simulink library "AD_Snowman_Library"  (R2023b)
settings: Solver=VariableStepAuto  StartTime=0.0  StopTime=10.0  RelTol=1e-3
libraries: simulink x1, $bdroot x1
settings Model: LastModifiedBy=USER

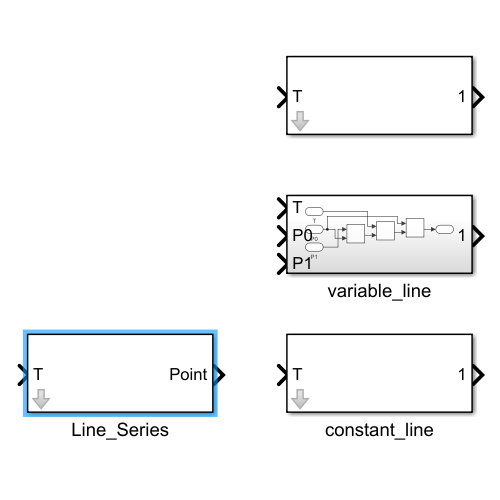
[thumbnail: Simulink's stored preview of the top-level diagram]
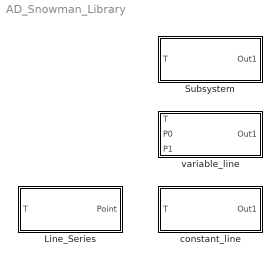
== system AD_Snowman_Library ==
  Line_Series : Subsystem  mask{PointMat=[0 0; 0 0]}
      mask prompts: PointMat "List of Points"
  Subsystem : Subsystem  mask{X_Offset=0, Y_Offset=0, A=0, B=0}
      mask prompts: X_Offset "X Offset"; Y_Offset "Y Offset"
      mask DialogControl DescTextVar Prompt: %<MaskDescription>A is the radius of X and B is the radius of Y
  constant_line : Subsystem  mask{P0=[0 0], P1=[0 0]}
      mask prompts: P0 "Start Point"; P1 "End Point"
  variable_line : Subsystem

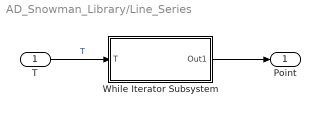
== system AD_Snowman_Library/Line_Series ==
  T : Inport
  While Iterator Subsystem : Subsystem  TreatAsAtomicUnit=on
  Point : Outport
  wires:
  T/1 -> While Iterator Subsystem/1(T)  "T"
  While Iterator Subsystem/1(Out1) -> Point/1

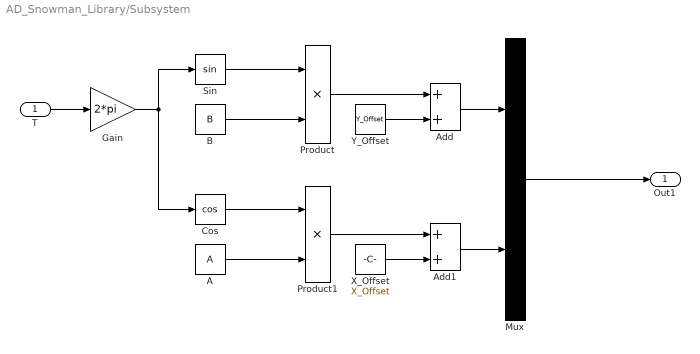
== system AD_Snowman_Library/Subsystem ==
  T : Inport
  A : Constant  Value=A
  Add : Sum
  Add1 : Sum
  B : Constant  Value=B
  Cos : Trigonometry  Operator=cos
  Gain : Gain  Gain=2*pi
  Mux : Mux  Inputs=2
  Product : Product
  Product1 : Product
  Sin : Trigonometry
  X_Offset : Constant  Value=X_Offset
  Y_Offset : Constant  Value=Y_Offset
  Out1 : Outport
  wires:
  Cos/1 -> Product1/1
  Sin/1 -> Product/1
  B/1 -> Product/2
  T/1 -> Gain/1
  A/1 -> Product1/2
  Add/1 -> Mux/1
  Add1/1 -> Mux/2
  X_Offset/1 -> Add1/2
  Product/1 -> Add/1
  Gain/1 -> Cos/1, Sin/1
  Product1/1 -> Add1/1
  Y_Offset/1 -> Add/2
  Mux/1 -> Out1/1

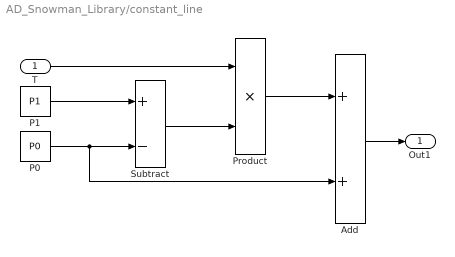
== system AD_Snowman_Library/constant_line ==
  T : Inport
  Add : Sum
  P0 : Constant  Value=P0
  P1 : Constant  Value=P1
  Product : Product
  Subtract : Sum  Inputs=+-
  Out1 : Outport
  wires:
  T/1 -> Product/1
  Subtract/1 -> Product/2
  Product/1 -> Add/1
  Add/1 -> Out1/1
  P0/1 -> Add/2, Subtract/2
  P1/1 -> Subtract/1

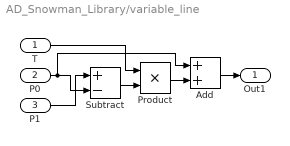
== system AD_Snowman_Library/variable_line ==
  T : Inport
  P0 : Inport  Port=2
  P1 : Inport  Port=3
  Add : Sum
  Product : Product
  Subtract : Sum  Inputs=+-
  Out1 : Outport
  wires:
  T/1 -> Product/1
  P0/1 -> Add/1, Subtract/2
  P1/1 -> Subtract/1
  Subtract/1 -> Product/2
  Product/1 -> Add/2
  Add/1 -> Out1/1

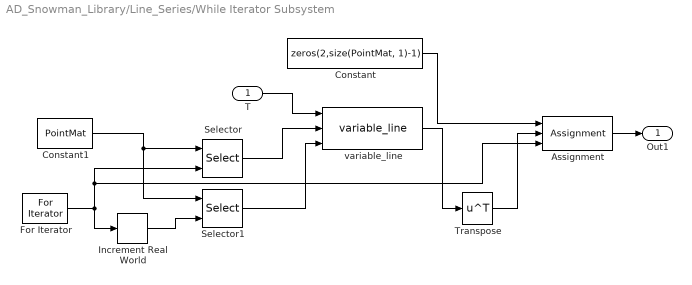
== system AD_Snowman_Library/Line_Series/While Iterator Subsystem ==
  T : Inport
  Assignment : Assignment  NumberOfDimensions=2  DiagnosticForDimensions=Warning  IndexOptions=Assign all,Index vector (port)  Indices=1,1  OutputSizes=1,1
  Constant : Constant  Value=zeros(2,size(PointMat, 1)-1)
  Constant1 : Constant  Value=PointMat
  For Iterator : ForIterator  IterationLimit=size(PointMat, 1)-1
  Increment Real World : simulink/Additional Math & Discrete/Additional Math: Increment - Decrement/Increment Real World
  Selector : Selector  NumberOfDimensions=2  InputPortWidth=3  IndexOptions=Index vector (port),Select all  Indices=[1 3],1  OutputSizes=1,1
  Selector1 : Selector  NumberOfDimensions=2  InputPortWidth=3  IndexOptions=Index vector (port),Select all  Indices=[1 3],1  OutputSizes=1,1
  Transpose : Math  Operator=transpose
  variable_line : $bdroot/variable_line  SystemSampleTime=-1  VariantActivationTime=update diagram  AllowFlexibleInterface=on  Latency=0  AutoFrameSizeCalculation=off
  Out1 : Outport
  wires:
  T/1 -> variable_line/1
  Constant/1 -> Assignment/1
  variable_line/1 -> Transpose/1
  Selector/1 -> variable_line/2
  Selector1/1 -> variable_line/3
  Constant1/1 -> Selector1/1, Selector/1
  For Iterator/1 -> Assignment/3, Selector/2, Increment Real World/1
  Increment Real World/1 -> Selector1/2
  Assignment/1 -> Out1/1
  Transpose/1 -> Assignment/2
